simulink model "combineBinnedDataFromArrays"  (R2012b)
settings: Solver=FixedStepDiscrete  StartTime=0.0  StopTime=10.0  FixedStep=0.001  RelTol=1e-3
settings Model: BufferReuse=off  Creator=gilja  LastModifiedBy=Chethan
settings SolverCC: EnableConcurrentExecution=on  ConcurrentTasks=on
settings DataIOCC: SaveOutput=off  SignalLogging=off  DSMLogging=off  SaveTime=off
settings OptimizationCC: InlineParams=on  InlineInvariantSignals=on  OptimizeBlockIOStorage=off  BufferReuse=off  ExpressionFolding=off  LocalBlockOutputs=off
settings HardwareCC: ProdIntDivRoundTo=Zero  ProdEndianess=LittleEndian  ProdHWDeviceType=Generic->32-bit x86 compatible
settings ModelReferenceCC: ModelReferenceMinAlgLoopOccurrences=on
settings RTWCC: SystemTargetFile=xpctarget.tlc  TemplateMakefile=xpc_default_tmf  Description=xPC Target  ProcessScript=xpctarget_make_rtw_hook  RTWCompilerOptimization=On
settings CodeAppCC: MaxIdLength=62
settings xpcTargetCC: TargetFcnLib=ansi_tfl_table_tmw.mat  CodeReplacementLibrary=XPC_BLAS  ParMdlRefBuildCompliant=on  ConcurrentExecutionCompliant=on  CombineSignalStateStructs=off  GRTInterface=on  xPCTaskExecutionProfile=on  xPCRL32EventNumber=5000  xPCisDownloadable=off  xPCLoadParamSetFile=off  xPCConcurrentTasks=off  xPCEnableSFAnimation=off

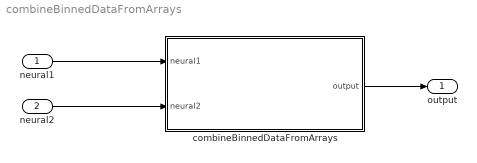
== system combineBinnedDataFromArrays ==
  neural1 : Inport
  neural2 : Inport  Port=2
  combineBinnedDataFromArrays : MATLAB Function  TreatAsAtomicUnit=on
  output : Outport  BusOutputAsStruct=on
  wires:
  combineBinnedDataFromArrays/1(output) -> output/1
  neural1/1 -> combineBinnedDataFromArrays/1(neural1)
  neural2/1 -> combineBinnedDataFromArrays/2(neural2)

== matlab function combineBinnedDataFromArrays/combineBinnedDataFromArrays ==
  data: neural1 input size=[1 uint16(2*DecoderConstants.NUM_CHANNELS_PER_ARRAY)]; neural2 input size=[1 uint16(2*DecoderConstants.NUM_CHANNELS_PER_ARRAY)]; output output
function output = combineBinnedDataFromArrays(neural1, neural2)
    persistent outputTmp
    if isempty(outputTmp)
        outputTmp = zeros([1, uint16(DecoderConstants.NUM_CONTINUOUS_CHANNELS)]);
    end
    
    % first put in the spike data
    outputTmp(1,(1:96)+(96*0)) = neural1(1,(1:96));
    outputTmp(1,(1:96)+(96*1)) = neural2(1,(1:96));
    
    % then add in lfp data
    outputTmp(1,(1:96)+(96*2)) = neural1(1,(1:96)+96);
    outputTmp(1,(1:96)+(96*3)) = neural2(1,(1:96)+96);

    output=outputTmp;
